simulink model "lqe_ins_h"  (R2020b)
settings: Solver=FixedStepDiscrete  StartTime=0.0  StopTime=10.0  RelTol=1e-3
settings Model: Creator=LEON  LastModifiedBy=leonk
settings DataIOCC: ReturnWorkspaceOutputs=off
settings OptimizationCC: DefaultParameterBehavior=Inlined  UseFloatMulNetSlope=on  InlineInvariantSignals=on  PassReuseOutputArgsAs=Individual arguments  ZeroExternalMemoryAtStartup=off  ZeroInternalMemoryAtStartup=off  NoFixptDivByZeroProtection=on  EfficientFloat2IntCast=on  LifeSpan=1  OptimizeBlockOrder=speed  DifferentSizesBufferReuse=on  EfficientTunableParamExpr=on
settings DebuggingCC: ParameterTunabilityLossMsg=error  ArithmeticOperatorsInVariantConditions=warning
settings HardwareCC: ProdBitPerPointer=32  ProdBitPerSizeT=32  ProdBitPerPtrDiffT=32  ProdWordSize=32  ProdLongLongMode=on  ProdHWDeviceType=Intel->x86-32 (Windows32)
settings SFSimCC: MATLABDynamicMemAlloc=off  CustomCodeUndefinedFunction=UseInterfaceOnly
settings RTWCC: Description=Embedded Coder  SystemTargetFile=ert.tlc  TemplateMakefile=ert_default_tmf  GenerateReport=on  IncludeHyperlinkInReport=on  LaunchReport=on  GenerateTraceInfo=on  GenerateTraceReport=on  GenerateTraceReportSl=on  GenerateTraceReportSf=on  GenerateTraceReportEml=on  GenerateCodeMetricsReport=on
settings CodeAppCC: ForceParamTrailComments=on  IgnoreCustomStorageClasses=off  OperatorAnnotations=on  SimulinkDataObjDesc=on  SFDataObjDesc=on  CustomSymbolStrGlobalVar=rt$N$M  CustomSymbolStrType=$N$M  CustomSymbolStrFcn=$N$M$F  CustomSymbolStrMacro=$N$M  InsertBlockDesc=on
settings ERTTargetCC: TargetLangStandard=C99 (ISO)  GenerateSampleERTMain=on  IncludeMdlTerminateFcn=off  CombineSignalStateStructs=on  SupportAbsoluteTime=off  SupportComplex=off  SupportNonInlinedSFcns=on  InlinedParameterPlacement=NonHierarchical  ERTCustomFileTemplate=example_file_process.tlc  ERTFilePackagingFormat=CompactWithDataFile

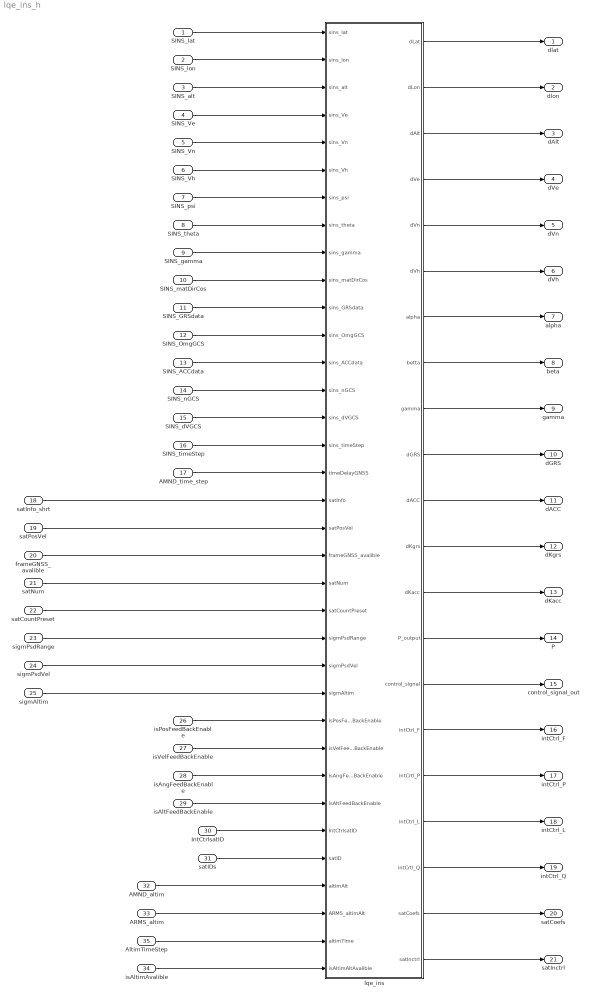
== system lqe_ins_h ==
  SINS_lat : Inport  PortDimensions=1
  SINS_lon : Inport  Port=2  PortDimensions=1
  SINS_alt : Inport  Port=3  PortDimensions=1
  SINS_Ve : Inport  Port=4  PortDimensions=1
  SINS_Vn : Inport  Port=5  PortDimensions=1
  SINS_Vh : Inport  Port=6  PortDimensions=1
  SINS_psi : Inport  Port=7  PortDimensions=1
  SINS_theta : Inport  Port=8  PortDimensions=1
  SINS_gamma : Inport  Port=9  PortDimensions=1
  SINS_matDirCos : Inport  Port=10  PortDimensions=[3,3]
  SINS_GRSdata : Inport  Port=11  PortDimensions=[3,1]
  SINS_OmgGCS : Inport  Port=12  PortDimensions=[3,1]
  SINS_ACCdata : Inport  Port=13  PortDimensions=[3,1]
  SINS_nGCS : Inport  Port=14  PortDimensions=[3,1]
  SINS_dVGCS : Inport  Port=15  PortDimensions=[3,1]
  SINS_timeStep : Inport  Port=16  PortDimensions=1
  AMND_time_step : Inport  Port=17  PortDimensions=1
  satInfo_shrt : Inport  Port=18  PortDimensions=[4,8]
  satPosVel : Inport  Port=19  PortDimensions=[6,8]
  frameGNSS_avalible : Inport  Port=20  OutDataTypeStr=uint8  PortDimensions=1
  satNum : Inport  Port=21  OutDataTypeStr=uint8  PortDimensions=1
  satCountPreset : Inport  Port=22  OutDataTypeStr=uint8  PortDimensions=1
  sigmPsdRange : Inport  Port=23  PortDimensions=8
  sigmPsdVel : Inport  Port=24  PortDimensions=8
  sigmAltim : Inport  Port=25  PortDimensions=1
  isPosFeedBackEnable : Inport  Port=26  OutDataTypeStr=uint8  PortDimensions=1
  isVelFeedBackEnable : Inport  Port=27  OutDataTypeStr=uint8  PortDimensions=1
  isAngFeedBackEnable : Inport  Port=28  OutDataTypeStr=uint8  PortDimensions=1
  isAltFeedBackEnable : Inport  Port=29  OutDataTypeStr=uint8  PortDimensions=1
  IntCtrlsatID : Inport  Port=30  OutDataTypeStr=uint8  PortDimensions=[3,1]
  satIDs : Inport  Port=31  OutDataTypeStr=uint8  PortDimensions=[8,1]
  AMND_altim : Inport  Port=32
  ARMS_altim : Inport  Port=33
  isAltimAvalible : Inport  Port=34
  AltimTimeStep : Inport  Port=35
  lqe_ins : MATLAB Function  TreatAsAtomicUnit=on
  dlat : Outport  PortDimensions=1  VectorParamsAs1DForOutWhenUnconnected=off
  dlon : Outport  Port=2  PortDimensions=1  VectorParamsAs1DForOutWhenUnconnected=off
  dAlt : Outport  Port=3  PortDimensions=1  VectorParamsAs1DForOutWhenUnconnected=off
  dVe : Outport  Port=4  PortDimensions=1  VectorParamsAs1DForOutWhenUnconnected=off
  dVn : Outport  Port=5  PortDimensions=1  VectorParamsAs1DForOutWhenUnconnected=off
  dVh : Outport  Port=6  PortDimensions=1  VectorParamsAs1DForOutWhenUnconnected=off
  alpha : Outport  Port=7  PortDimensions=1  VectorParamsAs1DForOutWhenUnconnected=off
  beta : Outport  Port=8  PortDimensions=1  VectorParamsAs1DForOutWhenUnconnected=off
  gamma : Outport  Port=9  PortDimensions=1  VectorParamsAs1DForOutWhenUnconnected=off
  dGRS : Outport  Port=10  PortDimensions=[3,1]  VectorParamsAs1DForOutWhenUnconnected=off
  dACC : Outport  Port=11  PortDimensions=[3,1]  VectorParamsAs1DForOutWhenUnconnected=off
  dKgrs : Outport  Port=12  PortDimensions=[3,1]  VectorParamsAs1DForOutWhenUnconnected=off
  dKacc : Outport  Port=13  PortDimensions=[3,1]  VectorParamsAs1DForOutWhenUnconnected=off
  P : Outport  Port=14  VectorParamsAs1DForOutWhenUnconnected=off
  control_signal_out : Outport  Port=15  PortDimensions=[4,1]  VectorParamsAs1DForOutWhenUnconnected=off
  intCtrl_F : Outport  Port=16  VectorParamsAs1DForOutWhenUnconnected=off
  intCtrl_P : Outport  Port=17  VectorParamsAs1DForOutWhenUnconnected=off
  intCtrl_L : Outport  Port=18  VectorParamsAs1DForOutWhenUnconnected=off
  intCtrl_Q : Outport  Port=19  VectorParamsAs1DForOutWhenUnconnected=off
  satCoefs : Outport  Port=20  PortDimensions=[4,3]  VectorParamsAs1DForOutWhenUnconnected=off
  satInctrl : Outport  Port=21  PortDimensions=3  VectorParamsAs1DForOutWhenUnconnected=off
  wires:
  SINS_lat/1 -> lqe_ins/1(sins_lat)
  SINS_lon/1 -> lqe_ins/2(sins_lon)
  SINS_Ve/1 -> lqe_ins/4(sins_Ve)
  SINS_Vn/1 -> lqe_ins/5(sins_Vn)
  SINS_Vh/1 -> lqe_ins/6(sins_Vh)
  SINS_psi/1 -> lqe_ins/7(sins_psi)
  SINS_theta/1 -> lqe_ins/8(sins_theta)
  SINS_gamma/1 -> lqe_ins/9(sins_gamma)
  SINS_matDirCos/1 -> lqe_ins/10(sins_matDirCos)
  SINS_GRSdata/1 -> lqe_ins/11(sins_GRSdata)
  SINS_OmgGCS/1 -> lqe_ins/12(sins_OmgGCS)
  SINS_ACCdata/1 -> lqe_ins/13(sins_ACCdata)
  SINS_nGCS/1 -> lqe_ins/14(sins_nGCS)
  AMND_time_step/1 -> lqe_ins/17(timeDelayGNSS)
  lqe_ins/15(control_signal) -> control_signal_out/1
  lqe_ins/14(P_output) -> P/1
  lqe_ins/13(dKacc) -> dKacc/1
  lqe_ins/12(dKgrs) -> dKgrs/1
  lqe_ins/11(dACC) -> dACC/1
  lqe_ins/10(dGRS) -> dGRS/1
  SINS_alt/1 -> lqe_ins/3(sins_alt)
  lqe_ins/1(dLat) -> dlat/1
  lqe_ins/2(dLon) -> dlon/1
  lqe_ins/3(dAlt) -> dAlt/1
  lqe_ins/4(dVe) -> dVe/1
  lqe_ins/5(dVn) -> dVn/1
  lqe_ins/6(dVh) -> dVh/1
  lqe_ins/7(alpha) -> alpha/1
  lqe_ins/8(betta) -> beta/1
  lqe_ins/9(gamma) -> gamma/1
  SINS_timeStep/1 -> lqe_ins/16(sins_timeStep)
  SINS_dVGCS/1 -> lqe_ins/15(sins_dVGCS)
  satInfo_shrt/1 -> lqe_ins/18(satInfo)
  satPosVel/1 -> lqe_ins/19(satPosVel)
  frameGNSS_avalible/1 -> lqe_ins/20(frameGNSS_avalible)
  satNum/1 -> lqe_ins/21(satNum)
  isPosFeedBackEnable/1 -> lqe_ins/26(isPosFeedBackEnable)
  isVelFeedBackEnable/1 -> lqe_ins/27(isVelFeedBackEnable)
  isAngFeedBackEnable/1 -> lqe_ins/28(isAngFeedBackEnable)
  isAltFeedBackEnable/1 -> lqe_ins/29(isAltFeedBackEnable)
  sigmPsdRange/1 -> lqe_ins/23(sigmPsdRange)
  sigmPsdVel/1 -> lqe_ins/24(sigmPsdVel)
  sigmAltim/1 -> lqe_ins/25(sigmAltim)
  satCountPreset/1 -> lqe_ins/22(satCountPreset)
  lqe_ins/16(intCtrl_F) -> intCtrl_F/1
  lqe_ins/17(intCrtl_P) -> intCtrl_P/1
  lqe_ins/18(intCtrl_L) -> intCtrl_L/1
  lqe_ins/19(intCrtl_Q) -> intCtrl_Q/1
  IntCtrlsatID/1 -> lqe_ins/30(IntCtrlsatID)
  satIDs/1 -> lqe_ins/31(satID)
  lqe_ins/20(satCoefs) -> satCoefs/1
  AMND_altim/1 -> lqe_ins/32(altimAlt)
  ARMS_altim/1 -> lqe_ins/33(ARMS_altimAlt)
  lqe_ins/21(satInctrl) -> satInctrl/1
  AltimTimeStep/1 -> lqe_ins/34(altimTime)
  isAltimAvalible/1 -> lqe_ins/35(isAltimAltAvalible)

== matlab function lqe_ins_h/lqe_ins ==
  data: sins_lat input; sins_lon input; sins_alt input; sins_Ve input; sins_Vn input; sins_Vh input; sins_psi input; sins_theta input; sins_gamma input; sins_matDirCos input; sins_GRSdata input; sins_OmgGCS input; sins_ACCdata input; sins_nGCS input; sins_dVGCS input; sins_timeStep input; timeDelayGNSS input; dLat output; dLon output; dAlt output; dVe output; dVn output; dVh output; alpha output; betta output; gamma output; dGRS output; dACC output; dKgrs output; dKacc output; P_output output; control_signal output; satInfo input; satPosVel input; frameGNSS_avalible input; satNum input; satCountPreset input; sigmPsdRange input; sigmPsdVel input; sigmAltim input; isPosFeedBackEnable input; isVelFeedBackEnable input; isAngFeedBackEnable input; isAltFeedBackEnable input; intCtrl_F output; intCrtl_P output; intCtrl_L output; intCrtl_Q output; IntCtrlsatID input; satID input; satCoefs output; satInctrl output; altimAlt input; ARMS_altimAlt input; altimTime input; isAltimAltAvalible input
function [dLat,dLon,dAlt,dVe,dVn,dVh,alpha,betta,gamma,dGRS, dACC, dKgrs,dKacc,...
    P_output, control_signal, intCtrl_F, intCrtl_P, intCtrl_L, intCrtl_Q, ...
    satCoefs, satInctrl]=...
    lqe_ins(...
    sins_lat, sins_lon, sins_alt, sins_Ve, sins_Vn, sins_Vh,sins_psi, sins_theta,...
    sins_gamma,sins_matDirCos, sins_GRSdata, sins_OmgGCS, sins_ACCdata,...
    sins_nGCS, sins_dVGCS,...
    sins_timeStep,...
    timeDelayGNSS,...
    satInfo, satPosVel, frameGNSS_avalible, satNum, satCountPreset,...
    sigmPsdRange, sigmPsdVel, sigmAltim,...
    isPosFeedBackEnable, isVelFeedBackEnable, isAngFeedBackEnable, isAltFeedBackEnable,...
    IntCtrlsatID, satID,...
    altimAlt, ARMS_altimAlt, altimTime,isAltimAltAvalible)

   
    persistent LQE SINS ready2resetFlag  %AMND 
    %---------------------------------------------
    %Constants
    u = deg2rad(15/3600); 
    EARTH_A = 6378147;
    EARTH_B = 6356751.3618;
    e2 = 0.0066943662;
    %Frequently used parameters
    
    RO_1 = EARTH_A*(1-e2)/(1-e2*sin(sins_lat)^2)^(3/2) + sins_alt;%EARTH_A;
    RO_2 = EARTH_A*(1-e2*sin(sins_lat)^2)^(-1/2) + sins_alt;%EARTH_A;
    GRAVIT_CONST_EATRH = 3.9860e+14;
    SQR_OM_SH = (GRAVIT_CONST_EATRH/(EARTH_A*EARTH_A*EARTH_A));
    
    %Предполагается контроль 3 сптуников. Так как уже заложена работа с 8-ю, а 5 спутников - минимум для контроля целостности 
    
    if isempty(LQE) 
        
        ready2resetFlag = 0;
        
        XSize_base     = 23;
        satInCtrl      = 3;
        satInCtrlMax   = 3;
        
        LQE.XSize_base   = XSize_base;
        LQE.satInCtrl    = satInCtrl;
        LQE.satInCtrlMax = 3;
        LQE.IntCtrlsatID = uint8(zeros(3,1));
        LQE.timeIntCtrl  = zeros(3,1);
        
        LQE.satID = uint8(zeros(8,1));
        LQE.IntCtrlsatCount = uint8(0);
        
        LQE.satIntCtrlNums = uint8(zeros(3,1));
       
       
        LQE.Z = zeros(                      17,                              1);
        LQE.X = zeros(XSize_base + satInCtrlMax*3,                           1);
        LQE.F = zeros(XSize_base + satInCtrlMax*3, XSize_base + satInCtrlMax*3);
        LQE.S = zeros(XSize_base + satInCtrlMax*3, XSize_base + satInCtrlMax*3);
        LQE.P = zeros(XSize_base + satInCtrlMax*3, XSize_base + satInCtrlMax*3);
        LQE.G = zeros(XSize_base + satInCtrlMax*3,                           6);
        LQE.L = zeros(XSize_base + satInCtrlMax*3,                           6);
        LQE.Q = zeros(                       6,                              6);
        LQE.K = zeros(XSize_base + satInCtrlMax*3,                          17);
        LQE.R = zeros(                      17,                             17);
        LQE.H = zeros(                      17,    XSize_base + satInCtrlMax*3);
        
        
        
        LQE.prediction_step     = sins_timeStep;
        LQE.isPosFeedBackEnable = isPosFeedBackEnable;%0;%
        LQE.isVelFeedBackEnable = isVelFeedBackEnable;%0;%
        LQE.isAngFeedBackEnable = isAngFeedBackEnable;%0;%
        LQE.isAltFeedBackEnable = isAltFeedBackEnable;
        
        LQE.isCrdCorrAvalible   = uint8(0);
        LQE.isVelCorrAvalible   = uint8(0);
        LQE.isAltGNSSAvalible   = uint8(0);
        LQE.isCorrAvalible      = uint8(0);
        
        LQE = init_PQ(LQE);
        
        SINS.lat   = 0;
        SINS.lon   = 0;
        SINS.alt   = 0;
        SINS.Ve    = 0;
        SINS.Vn    = 0;
        SINS.Vh    = 0;
        SINS.psi   = 0;
        SINS.theta = 0;
        SINS.gamma = 0;
        SINS.matDirCos = zeros(3,3);
        SINS.Omg_x = 0;
        SINS.Omg_y = 0;
        SINS.Omg_z = 0;
        SINS.Omg_e = 0;
        SINS.Omg_n = 0;
        SINS.Omg_h = 0;
        SINS.n_x   = 0;
        SINS.n_y   = 0;
        SINS.n_z   = 0;
        SINS.n_e   = 0;
        SINS.n_n   = 0;
        SINS.n_h   = 0;
        SINS.dV_e  = 0;
        SINS.dV_n  = 0;
        SINS.dV_h  = 0;
        
    end 

    lqeIndexes = 1 : 1 : LQE.XSize_base + LQE.satInCtrl*3;  

    if frameGNSS_avalible == 1 && any(IntCtrlsatID ~= 0)       
        LQE.timeIntCtrl = LQE.timeIntCtrl + timeDelayGNSS;
        if all(LQE.IntCtrlsatID == 0)
            ready2resetFlag = 1;
        else
            ready2resetFlag = 0;
        end

        LQE.satID =             satID;
        satPosBanned =          [0,0,0];
        timeIntCtrl =           zeros(3,1);
        timeIntCtrl =           LQE.timeIntCtrl;
        LQE.timeIntCtrl =       zeros(3,1);
        P_save =                zeros(9,1);
        P_save =                diag(LQE.P(24:end,24:end));
        X_save =                zeros(9,1);
        X_save =                LQE.X(24:end);
        LQE.X(24:end)   =       0;
        LQE.P(24:end,:) =       0;
        LQE.P(:,24:end) =       0;
        LQE.P(24:end,24:end) =  diag(ones(9,1) .* 1e-8);
    %Если спутники были
    %Спутников не болше чем на контроле
    %Спутники отсортированы по номерам ID


        for ii = 1:LQE.satInCtrl
             if IntCtrlsatID(ii)~= 0
                LQE.satIntCtrlNums(ii) = find(IntCtrlsatID(ii) == LQE.satID); %Найти номер чертовского спутника в листе всех
                satIntCtrlID = find(IntCtrlsatID(ii) == LQE.IntCtrlsatID);%Был ли спутник на контроле, то под каким номером из трёх
        
                
                if length(satIntCtrlID) ~= 0 %%&& ready2resetFlag == 0%Если был
                    satPosBanned(ii) = 1;
                    jj = satIntCtrlID(1,1);
                    LQE.timeIntCtrl(jj) = timeIntCtrl(ii);
                    
                    if ready2resetFlag == 0
                        LQE.P(23 + (ii-1)*3 + 1, 23 + (ii-1)*3 + 1) = P_save((jj-1)*3 + 1,1);
                        LQE.P(23 + (ii-1)*3 + 2, 23 + (ii-1)*3 + 2) = P_save((jj-1)*3 + 2,1);
                        LQE.P(23 + (ii-1)*3 + 3, 23 + (ii-1)*3 + 3) = P_save((jj-1)*3 + 3,1);
                    else
                        LQE.timeIntCtrl(ii) = 0;
                        LQE.P(23 + (ii-1)*3 + 1, 23 + (ii-1)*3 + 1) =  5^2;
                        LQE.P(23 + (ii-1)*3 + 2, 23 + (ii-1)*3 + 2) =  5^2;
                        LQE.P(23 + (ii-1)*3 + 3, 23 + (ii-1)*3 + 3) =  5^2;
                    end
                    
                    LQE.X(23 + (ii-1)*3 + 1,1) = X_save((jj-1)*3 + 1,1);
                    LQE.X(23 + (ii-1)*3 + 2,1) = X_save((jj-1)*3 + 2,1);
                    LQE.X(23 + (ii-1)*3 + 3,1) = X_save((jj-1)*3 + 3,1);
                else

                    LQE.timeIntCtrl(ii) = 0;
                    LQE.P(23 + (ii-1)*3 + 1, 23 + (ii-1)*3 + 1) =  5^2;
                    LQE.P(23 + (ii-1)*3 + 2, 23 + (ii-1)*3 + 2) =  5^2;
                    LQE.P(23 + (ii-1)*3 + 3, 23 + (ii-1)*3 + 3) =  5^2;
                end
            end 
            LQE.IntCtrlsatID = IntCtrlsatID;
         end
     end
        
%Определение размерности выходных данных
    dLat = 0; dLon = 0; dVe = 0; dVn = 0; alpha = 0; betta = 0; gamma = 0;
    dGRS=zeros(3,1); dACC=zeros(3,1); dKgrs=zeros(3,1); dKacc=zeros(3,1);
    
    P_output = zeros(length(LQE.P),1);
    
    intCtrl_F = zeros(length(LQE.F),length(LQE.F));
    intCrtl_P = zeros(length(LQE.P),length(LQE.P));
    intCtrl_L = zeros(size(LQE.L));
    intCrtl_Q = zeros(size(LQE.Q));
    intCrtl_Z = zeros(size(LQE.Z));
    
    satCoefs = zeros(4,3);
    satInctrl      = uint8(zeros(3,1));
    control_signal = zeros(4,1);
%%%%%%%%%%%%%%%%%%%%%%%%%%%%%%%%%%%%%%%%%%%%%%%%%%%%%%%%%%%%%%%%%%%%%%%%%%%    
    LQE.isPosFeedBackEnable = isPosFeedBackEnable;
    LQE.isVelFeedBackEnable = isVelFeedBackEnable;
    LQE.isAngFeedBackEnable = isAngFeedBackEnable;
    LQE.isAltFeedBackEnable = isAltFeedBackEnable;
    
    LQE.isCorrAvalible      = frameGNSS_avalible;
    LQE.isCorrAvalible = uint8(0);
    if frameGNSS_avalible == 1 || isAltimAltAvalible == 1
        LQE.isCorrAvalible = uint8(1);
    end
    
    SINS = parse_SINS(SINS, sins_lat, sins_lon, sins_alt, sins_Ve, sins_Vn,sins_Vh,...
        sins_psi, sins_theta, sins_gamma,...
        sins_matDirCos, sins_GRSdata, sins_OmgGCS, sins_ACCdata,sins_nGCS, sins_dVGCS);
                    
    LQE = update_GFL(LQE, SINS, RO_1, RO_2, u, SQR_OM_SH);
    
    % Прогноз
    LQE.X(lqeIndexes,:) = LQE.F(lqeIndexes,lqeIndexes)*LQE.X(lqeIndexes,:); 
    LQE.S(lqeIndexes,lqeIndexes) = LQE.F(lqeIndexes,lqeIndexes)*LQE.P(lqeIndexes,lqeIndexes)*LQE.F(lqeIndexes,lqeIndexes)' + LQE.L(lqeIndexes,:)*LQE.Q*LQE.L(lqeIndexes,:)';

    %Коррекция
    
    if LQE.isCorrAvalible == 1 
    
      LQE.Z = zeros(17,1);
      if frameGNSS_avalible == 1 
        LQE.Z(1:8)  = satInfo(2,:);
        LQE.Z(9:16) = satInfo(3,:);
      end    
      if isAltimAltAvalible == 1
        LQE.Z(17)   = SINS.alt - altimAlt;
      end
        %------------------------------------------------------------------
        LQE = update_H(LQE, SINS, RO_1, RO_2, EARTH_A, EARTH_B, e2, satInfo, satPosVel, satNum, satCountPreset, frameGNSS_avalible, isAltimAltAvalible); %Матрица H
        LQE = update_R(LQE, satNum, satCountPreset, timeDelayGNSS, sigmPsdRange, sigmPsdVel, ARMS_altimAlt, altimTime, frameGNSS_avalible, isAltimAltAvalible);
        %------------------------------------------------------------------
        LQE.K(lqeIndexes,:) = (LQE.S(lqeIndexes,lqeIndexes)*LQE.H(:,lqeIndexes)')*inv(LQE.H(:,lqeIndexes)*LQE.S(lqeIndexes,lqeIndexes)*LQE.H(:,lqeIndexes)' + LQE.R);
        LQE.P(lqeIndexes,lqeIndexes) = (eye(size(LQE.P(lqeIndexes,lqeIndexes))) - LQE.K(lqeIndexes,:)*LQE.H(:,lqeIndexes))*LQE.S(lqeIndexes,lqeIndexes);
        LQE.X(lqeIndexes,:) = LQE.X(lqeIndexes,:) + LQE.K(lqeIndexes,:)*(LQE.Z - LQE.H(:,lqeIndexes)*LQE.X(lqeIndexes,:));
    else
        LQE.P(lqeIndexes,lqeIndexes) = LQE.S(lqeIndexes,lqeIndexes);
    end 
    
    if LQE.P(1,1)   < (0.1^2) LQE.P(1,1)   = 0.1^2; end
    if LQE.P(2,2)   < (0.1^2) LQE.P(2,2)   = 0.1^2; end
    if LQE.P(20,20) < (0.1^2) LQE.P(20,20) = 0.1^2; end
    
    if LQE.P(3,3)   < (0.1^2) LQE.P(3,3)   = 0.1^2; end
    if LQE.P(4,4)   < (0.1^2) LQE.P(4,4)   = 0.1^2; end
    if LQE.P(21,21) < (0.1^2) LQE.P(21,21) = 0.1^2; end
    
    
    if LQE.P(24,24) < (0.1^2)   LQE.P(24,24)   = 0.1^2; end
    if LQE.P(25,25) < (0.1^2)   LQE.P(25,25)   = 0.1^2; end
    if LQE.P(26,26) < (0.1^2)   LQE.P(26,26)   = 0.1^2; end
    
    if LQE.P(27,27) < (0.1^2)   LQE.P(27,27)   = 0.1^2; end
    if LQE.P(28,28) < (0.1^2)   LQE.P(28,28)   = 0.1^2; end
    if LQE.P(29,29) < (0.1^2)   LQE.P(29,29)   = 0.1^2; end
    
    if LQE.P(30,30) < (0.1^2)   LQE.P(30,30)   = 0.1^2; end
    if LQE.P(31,31) < (0.1^2)   LQE.P(31,31)   = 0.1^2; end
    if LQE.P(32,32) < (0.1^2)   LQE.P(32,32)   = 0.1^2; end
    
    
    [dLat,dLon,dAlt,dVe,dVn,dVh,alpha,betta,gamma,dGRS,dACC,dKgrs,dKacc,P_output,...
                  LQE, control_signal,satCoefs,satInctrl] = parse_back(LQE,SINS,EARTH_A);
  
    intCtrl_F = LQE.F;
    intCrtl_P = LQE.P;
    intCtrl_L = LQE.L;
    intCrtl_Q = LQE.Q;
    intCrtl_Z = LQE.Z;
    
    
end
%=============================================================================================================
function LQE = update_R(LQE, satNum, satCountPreset, timeDelayGNSS, sigmPsdRange, sigmPsdVel, ARMS_altimAlt, altimTime, frameGNSS_avalible, isAltimAltAvalible)

    if frameGNSS_avalible == 1
        for ii = 1:satCountPreset
            if ii <= satNum
                LQE.R(ii,ii)                                    = (sigmPsdRange(ii).^2) / timeDelayGNSS;
                LQE.R(satCountPreset + ii, satCountPreset + ii) = (sigmPsdVel(ii).^2  ) / timeDelayGNSS;
            else 
                LQE.R(ii,ii)                                    = (10^2)              / timeDelayGNSS;
                LQE.R(satCountPreset + ii, satCountPreset + ii) = (10^2)              / timeDelayGNSS;
            end 

        end
    else
        LQE.R(1:16, 1:16) = eye(16) .*10000;
    end    
    
    if isAltimAltAvalible == 1
        LQE.R(17, 17) = (ARMS_altimAlt^2) / altimTime;
    else 
        LQE.R(17, 17) = 10000;
    end
end
%=============================================================================================================
function LQE = update_H(LQE, SINS, ro_1, ro_2, a, b, e2, satInfo, satPosVel, satNum, satCountPreset, frameGNSS_avalible, isAltimAltAvalible)


    LQE.H = zeros(size(LQE.H));

    if isAltimAltAvalible == 1
        LQE.H(17, 20) = 1;
    end
    if frameGNSS_avalible == 1
        posObj = zeros(3,1);

        Rz = (a) ./ sqrt(1-e2*(sin(SINS.lat).^2));

        dRz_dLat = a*e2*cos(SINS.lat)*sin(SINS.lat) / ((1 - e2*sin(SINS.lat)^2)^(3/2));
        R_tp     = sin(SINS.lat)*(Rz + SINS.alt) - cos(SINS.lat)*dRz_dLat;     

        posObj(1) = (Rz + SINS.alt)*cos(SINS.lat)*cos(SINS.lon);
        posObj(2) = (Rz + SINS.alt)*cos(SINS.lat)*sin(SINS.lon);
        posObj(3) = (((b^2)/(a^2))*Rz + SINS.alt)*sin(SINS.alt);

        for ii = 1:satCountPreset 
            if ii <= satNum


                dPsdRange_dLambda = (1/satInfo(4,ii))* (Rz + SINS.alt)*cos(SINS.lat)*...
                   (sin(SINS.lon)*(satPosVel(1,ii) - posObj(1)) - ...
                    cos(SINS.lon)*(satPosVel(2,ii) - posObj(2)));% * d_lon; % d_lon???

                dPsdRange_dphi = (1 / satInfo(4,ii)) * ...
                        ((satPosVel(1,ii) - posObj(1)) * (- cos(SINS.lon) * cos(SINS.lat) * R_tp + (Rz + SINS.alt) * cos(SINS.lon) * sin(SINS.lat)) + ...%dRz_dLat
                         (satPosVel(2,ii) - posObj(2)) * (- sin(SINS.lon) * cos(SINS.lat) * R_tp + (Rz + SINS.alt) * sin(SINS.lon) * sin(SINS.lat)) + ...%dRz_dLat
                         (satPosVel(3,ii) - posObj(3)) * (- (1 - e2)      * sin(SINS.lat) * R_tp - ((1 - e2) * Rz + SINS.alt)      * cos(SINS.lat)));    %dRz_dLat


                dPsdVel_dot_dVe   = (1/satInfo(4,ii)) * (...
                    sin(SINS.lon) * (satPosVel(1,ii) - posObj(1)) - ...
                    cos(SINS.lon) * (satPosVel(2,ii) - posObj(2)));% * d_Ve;

                dPsdVel_dot_dVn   =  (1/satInfo(4,ii)) * (...
                    cos(SINS.lon)*sin(SINS.lat)*(satPosVel(1,ii) - posObj(1)) + ...
                    sin(SINS.lon)*sin(SINS.lat)*(satPosVel(2,ii) - posObj(2)) - ...
                    cos(SINS.lat)*              (satPosVel(3,ii) - posObj(3)));%*d_Vn;

                dPsdRange_dAlt    = (-1/satInfo(4,ii))* (...
                    cos(SINS.lat)*cos(SINS.lon)*(satPosVel(1,ii) - posObj(1)) + ...
                    cos(SINS.lat)*sin(SINS.lon)*(satPosVel(2,ii) - posObj(2)) + ...
                    sin(SINS.lat)*              (satPosVel(3,ii) - posObj(3)));%*d_alt;

                dPsdVel_dot_dVh = (-1/satInfo(4,ii))* (...
                    cos(SINS.lon)*cos(SINS.lat)*(satPosVel(1,ii) - posObj(1)) + ...
                    sin(SINS.lon)*cos(SINS.lat)*(satPosVel(2,ii) - posObj(2)) + ...
                    sin(SINS.lat)*              (satPosVel(3,ii) - posObj(3)));%*d_vh;


                LQE.H(ii,1) =  (1/(ro_2 * cos(SINS.lat))) * dPsdRange_dLambda;%longitude
                LQE.H(ii,2) =  (1/ro_1) * dPsdRange_dphi;%latitude
                LQE.H(ii,20)=  dPsdRange_dAlt;% altitude Было 22

                LQE.H(ii,22)= -1;%delta t Было 20, стало 22 (вертикальный канал 19 и 20)

                LQE.H(satCountPreset + ii,1) = - (SINS.Vh/ro_2 + SINS.Omg_e*tan(SINS.lat)) * dPsdVel_dot_dVe;%Перенесено в ii - 2 - (SINS.Vh/ro_1)*dPsdVel_dot_dVn;
                LQE.H(satCountPreset + ii,2) = - SINS.Omg_h * dPsdVel_dot_dVe - (SINS.Vh/ro_1)*dPsdVel_dot_dVn;
                LQE.H(satCountPreset + ii,20)=   SINS.Omg_n * dPsdVel_dot_dVe - SINS.Omg_e*dPsdVel_dot_dVn;%Добавлено от Савкина

                LQE.H(satCountPreset + ii,3) =   dPsdVel_dot_dVe;
                LQE.H(satCountPreset + ii,4) =   dPsdVel_dot_dVn;
                LQE.H(satCountPreset + ii,21)=   dPsdVel_dot_dVh; % Vh       Было 23
                LQE.H(satCountPreset + ii,23)=   1;
            end
        end
        for ii = 0:LQE.satInCtrlMax - 1
                if LQE.IntCtrlsatID(ii+1) ~= 0
                    LQE.H(LQE.satIntCtrlNums(ii+1), 23 + (ii*3) + 1) =  -1;
                    LQE.H(LQE.satIntCtrlNums(ii+1), 23 + (ii*3) + 2) =  -LQE.timeIntCtrl(ii + 1);
                    LQE.H(LQE.satIntCtrlNums(ii+1), 23 + (ii*3) + 3) =  -(LQE.timeIntCtrl(ii + 1)^2);
                end
        end 
    end

end



%==========================================================================

function LQE = init_PQ(LQE)

    GRS_noise = deg2rad(0.15*1e-5)/60;
    ACC_noise = 1e-5;
    LQE.Q = diag([GRS_noise;GRS_noise;GRS_noise;... 
                    ACC_noise;ACC_noise;ACC_noise].^2)/LQE.prediction_step;
%     setv new 14:27 22.03.2021
    
    LQE.P = diag([10;10;0.77;0.77;...                                      %lon,lat,Ve,Vn
                  deg2rad(0.03);deg2rad(0.03);deg2rad(0.25);...            %alpha, betta, gamma
                  1.5*1e-5;1.5*1e-5;1.5*1e-5;...                           %dGRS
                  5*1e-3;5*1e-3;5*1e-3;...                                 %dKrgs
                  0.004;0.004;0.004;...                                    %dACC
                  3*1e-4;3*1e-4;3*1e-4;...                                 %dKacc
                  5;0.06; ...                                              %alt, Vh
                  1e-9; 1e-9;...                                           %dt, dt_dor
                  ones(3*3,1) * 1e-8].^2);                                 %sat coefs 

                             
end
%==========================================================================
function [dLat,dLon,dAlt,dVe,dVn,dVh,alpha,betta,gamma,dGRS, dACC, dKgrs,dKacc,...
             P_output, LQE, control_signal, satCoefs, satInctrl] = parse_back(LQE,SINS,EARTH_A) %AMND
  
    dLon  = LQE.X(1,1)/(EARTH_A*cos(SINS.lat));                            %d_longitude
    dLat  = LQE.X(2,1)/(EARTH_A);                                          %d_latitude
    dAlt  = LQE.X(20,1);%%%%%%%%%%%%%%%%%%%%%%%%%%%%%%%%%%%%%%%%%%
    dVe   = LQE.X(3,1) - tan(SINS.lat)*dLon*LQE.X(1,1) - SINS.Omg_h*LQE.X(2,1);%d_Ve
    dVn   = LQE.X(4,1);                                                    %d_Vn
    dVh   = LQE.X(21,1);%%%%%%%%%%%%%%%%%%
    alpha = LQE.X(5,1) + (1/EARTH_A)*LQE.X(2);                             %d_alpha
    betta = LQE.X(6,1) - (1/EARTH_A)*LQE.X(1);                             %d_betta
    gamma = LQE.X(7,1) - (1/EARTH_A)*LQE.X(1)*tan(SINS.lat);               %d_gamma
    dGRS  = [LQE.X(8:10)];
    dKgrs = [LQE.X(11:13)];
    dACC  = [LQE.X(14:16)];
    dKacc = [LQE.X(17:19)];
        
    P_output = sqrt(diag(LQE.P));
    
    control_signal = zeros(4,1);
    if  (LQE.isPosFeedBackEnable == 1) && (LQE.isCorrAvalible == 1)
        LQE.X(1)  = 0;
        LQE.X(2)  = 0;
        control_signal(1) = 1;
    end
    if  (LQE.isVelFeedBackEnable == 1) && (LQE.isCorrAvalible == 1)
        LQE.X(3)  = 0;
        LQE.X(4)  = 0;
        control_signal(2) = 1;
    end
    if  (LQE.isAngFeedBackEnable == 1) && (LQE.isCorrAvalible == 1)
        LQE.X(5) = 0;
        LQE.X(6) = 0;
        LQE.X(7) = 0;
        control_signal(3) = 1;
    end
    if  (LQE.isAltFeedBackEnable == 1) && (LQE.isCorrAvalible == 1)
        LQE.X(20) = 0;       
        LQE.X(21) = 0;
        control_signal(4) = 1;
    end  
    
    
    satCoefs      = zeros(4,3);
    satInctrl     = zeros(1,3);
    
    
    satCoefs(:,1) = [LQE.X(24:26) ; LQE.timeIntCtrl(1)];
    satCoefs(:,2) = [LQE.X(27:29) ; LQE.timeIntCtrl(2)];
    satCoefs(:,3) = [LQE.X(30:32) ; LQE.timeIntCtrl(3)];
    satInctrl     = LQE.IntCtrlsatID;
end
%==========================================================================

%==========================================================================
function LQE = update_GFL(LQE, SINS, RO_1, RO_2, u, omg_0)

    LQE.F = zeros(size(LQE.F));
    LQE.L = zeros(size(LQE.L));
    
    omg_e_dot = (-1/RO_1)*(SINS.dV_n - SINS.Vh*SINS.Vn/RO_1);
    omg_n_dot = (1/RO_2)*(SINS.dV_e - u*sin(SINS.lat)*SINS.Vn - SINS.Vh*SINS.Ve/RO_2);
    Omg_h_dot =1/RO_2*(u*cos(SINS.lat)*SINS.Ve + SINS.n_e*tan(SINS.lat)+...
           + SINS.Vh*SINS.Omg_h + SINS.Ve*SINS.Vn/(RO_2*cos(SINS.lat).^2));
       
    LQE.G(3,4) = SINS.matDirCos(1,1);
    LQE.G(3,5) = SINS.matDirCos(1,2);
    LQE.G(3,6) = SINS.matDirCos(1,3);
    
    LQE.G(4,4) = SINS.matDirCos(2,1);
    LQE.G(4,5) = SINS.matDirCos(2,2);
    LQE.G(4,6) = SINS.matDirCos(2,3);
    
    LQE.G(21,4) = SINS.matDirCos(3,1);%%%%%%%%%%%%%%%%%%%%%%%%%%%%%%
    LQE.G(21,5) = SINS.matDirCos(3,2);%%%%%%%%%%%%%%%%%%%%%%%%%%%%%%
    LQE.G(21,6) = SINS.matDirCos(3,3);%%%%%%%%%%%%%%%%%%%%%%%%%%%%%%
    
    LQE.G(5,1) = SINS.matDirCos(1,1);
    LQE.G(5,2) = SINS.matDirCos(1,2);
    LQE.G(5,3) = SINS.matDirCos(1,3);
    
    LQE.G(6,1) = SINS.matDirCos(2,1);
    LQE.G(6,2) = SINS.matDirCos(2,2);
    LQE.G(6,3) = SINS.matDirCos(2,3);

    LQE.G(7,1) = SINS.matDirCos(3,1);
    LQE.G(7,2) = SINS.matDirCos(3,2);
    LQE.G(7,3) = SINS.matDirCos(3,3);
         
    LQE.F(1,3) = 1; 
    LQE.F(2,4) = 1;
    
    LQE.F(3,1) = -omg_0.^2  + SINS.Omg_n.^2+SINS.Omg_h.^2;
    LQE.F(3,2) =  Omg_h_dot - SINS.Omg_e*SINS.Omg_n;
    LQE.F(3,4) =  2*SINS.Omg_h;
    
    LQE.F(4,1) = - LQE.F(3,2);
    LQE.F(4,2) = -omg_0.^2 + SINS.Omg_e.^2+SINS.Omg_h.^2;
    LQE.F(4,3) = -LQE.F(3,4);   

%     LQE.F(3,6)  = -SINS.n_h;% 
%     LQE.F(3,7)  =  SINS.n_n;% 
%     LQE.F(4,5)  =  SINS.n_h;% 
%     LQE.F(4,7)  = -SINS.n_e;% 
%     LQE.F(21,5) = -SINS.n_n;%%%%%%%%%%%%%%%%%%
%     LQE.F(21,6) =  SINS.n_e;%%%%%%%%%%%%%%%%%%%

    LQE.F(3,6)  =  SINS.n_h;% 
    LQE.F(3,7)  = -SINS.n_n;% 
    LQE.F(4,5)  = -SINS.n_h;% 
    LQE.F(4,7)  =  SINS.n_e;% 
    LQE.F(21,5) =  SINS.n_n;%%%%%%%%%%%%%%%%%%
    LQE.F(21,6) = -SINS.n_e;%%%%%%%%%%%%%%%%%%%

    
    
    LQE.F(5,5) =  0;
    LQE.F(5,6) =  SINS.Omg_h;%z
    LQE.F(5,7) = -SINS.Omg_n;%y
    
    LQE.F(6,5) = -SINS.Omg_h;%z
    LQE.F(6,6) =  0;
    LQE.F(6,7) =  SINS.Omg_e;%x
    
    LQE.F(7,5) =  SINS.Omg_n;%y%%%%%%%%%%%%%%%%%%%%%SINS.Omg_n
    LQE.F(7,6) = -SINS.Omg_e;%x
    LQE.F(7,7) =  0;
   
    LQE.F(5,8)   = SINS.matDirCos(1,1);
    LQE.F(5,9)   = SINS.matDirCos(1,2);
    LQE.F(5,10)  = SINS.matDirCos(1,3);
    
    LQE.F(6,8)   = SINS.matDirCos(2,1);
    LQE.F(6,9)   = SINS.matDirCos(2,2);
    LQE.F(6,10)  = SINS.matDirCos(2,3);
    
    LQE.F(7,8)   = SINS.matDirCos(3,1);
    LQE.F(7,9)   = SINS.matDirCos(3,2);
    LQE.F(7,10)  = SINS.matDirCos(3,3);
    
    LQE.F(5,11)   = SINS.Omg_x*SINS.matDirCos(1,1);
    LQE.F(5,12)   = SINS.Omg_y*SINS.matDirCos(1,2);
    LQE.F(5,13)   = SINS.Omg_z*SINS.matDirCos(1,3);
    
    LQE.F(6,11)   = SINS.Omg_x*SINS.matDirCos(2,1);
    LQE.F(6,12)   = SINS.Omg_y*SINS.matDirCos(2,2);
    LQE.F(6,13)   = SINS.Omg_z*SINS.matDirCos(2,3);
    
    LQE.F(7,11)   = SINS.Omg_x*SINS.matDirCos(3,1);
    LQE.F(7,12)   = SINS.Omg_y*SINS.matDirCos(3,2);
    LQE.F(7,13)   = SINS.Omg_z*SINS.matDirCos(3,3);
    
    LQE.F(3,14) = SINS.matDirCos(1,1);
    LQE.F(3,15) = SINS.matDirCos(1,2);
    LQE.F(3,16) = SINS.matDirCos(1,3);
    
    LQE.F(4,14) = SINS.matDirCos(2,1);
    LQE.F(4,15) = SINS.matDirCos(2,2);
    LQE.F(4,16) = SINS.matDirCos(2,3);
    
    LQE.F(3,17) = SINS.n_x*SINS.matDirCos(1,1);
    LQE.F(3,18) = SINS.n_y*SINS.matDirCos(1,2);
    LQE.F(3,19) = SINS.n_z*SINS.matDirCos(1,3);
    
    LQE.F(4,17) = SINS.n_x*SINS.matDirCos(2,1);
    LQE.F(4,18) = SINS.n_y*SINS.matDirCos(2,2);
    LQE.F(4,19) = SINS.n_z*SINS.matDirCos(2,3);

    LQE.F(3,20) = -(omg_n_dot + SINS.Omg_e*SINS.Omg_h);%%%%%%%%%%%%%%%%%%%%%%
    LQE.F(3,21) = -2*SINS.Omg_n;                       %%%%%%%%%%%%%%%%%%%%%% 
    
    LQE.F(4,20) = omg_e_dot - SINS.Omg_n*SINS.Omg_h;%%%%%%%%%%%%%%%%%%%%%%%%%%%%%
    LQE.F(4,21) = 2*SINS.Omg_e;
    
    LQE.F(20,21) = 1;
    
    LQE.F(21,1)  =  omg_n_dot -SINS.Omg_e*SINS.Omg_h; 
    LQE.F(21,3)  =  2*SINS.Omg_n;
    LQE.F(21,2)  = -(omg_e_dot + SINS.Omg_n*SINS.Omg_h);
    LQE.F(21,4)  =  2*SINS.Omg_e;

    LQE.F(21,14) = SINS.matDirCos(3,1);
    LQE.F(21,15) = SINS.matDirCos(3,2);
    LQE.F(21,16) = SINS.matDirCos(3,3);
    
    LQE.F(21,17) = SINS.n_x*SINS.matDirCos(3,1);
    LQE.F(21,18) = SINS.n_y*SINS.matDirCos(3,2);
    LQE.F(21,19) = SINS.n_z*SINS.matDirCos(3,3);
    
    LQE.F(21,20) =  2*omg_0.^2 + SINS.Omg_e.^2 + SINS.Omg_n.^2;%&&&&&&&&&&&&&&&&&&&&&&&  
    
    LQE.F = eye(size(LQE.F)) + LQE.F.*LQE.prediction_step;% + (1/2)*LQE.F^2.*LQE.prediction_step;
    LQE.L = LQE.F*LQE.G.*LQE.prediction_step;
end
%==========================================================================
function SINS = parse_SINS(SINS, sins_lat, sins_lon, sins_alt, sins_Ve, sins_Vn,sins_Vh,...
         sins_psi, sins_theta, sins_gamma,...
         sins_matDirCos, sins_GRSdata, sins_OmgGCS, sins_ACCdata,sins_nGCS,sins_dVGCS)

	SINS.lat   = sins_lat;
    SINS.lon   = sins_lon;
    SINS.alt   = sins_alt;
    SINS.Ve    = sins_Ve;
    SINS.Vn    = sins_Vn;
    SINS.Vh    = sins_Vh;
    SINS.psi   = sins_psi;
    SINS.theta = sins_theta;
    SINS.gamma = sins_gamma;
    SINS.matDirCos = sins_matDirCos;
    
    SINS.Omg_x = sins_GRSdata(1);
    SINS.Omg_y = sins_GRSdata(2);
    SINS.Omg_z = sins_GRSdata(3);
    
    SINS.Omg_e = sins_OmgGCS(1);
    SINS.Omg_n = sins_OmgGCS(2);
    SINS.Omg_h = sins_OmgGCS(3);
    
    SINS.n_x = sins_ACCdata(1);
    SINS.n_y = sins_ACCdata(2);
    SINS.n_z = sins_ACCdata(3);
    
    SINS.n_e = sins_nGCS(1);
    SINS.n_n = sins_nGCS(2);
    SINS.n_h = sins_nGCS(3);
    
    SINS.dV_e = sins_dVGCS(1);
    SINS.dV_n = sins_dVGCS(2);
    SINS.dV_h = sins_dVGCS(3);
    
end
